simulink model "Drone_Video_Test"  (R2024a)
settings: Solver=FixedStepAuto  StartTime=0.0  StopTime=inf  RelTol=1e-3
undefined symbols (not defined in the file or in its folder): VideoDirection
settings Model: Creator=Sasha  LastModifiedBy=Sasha

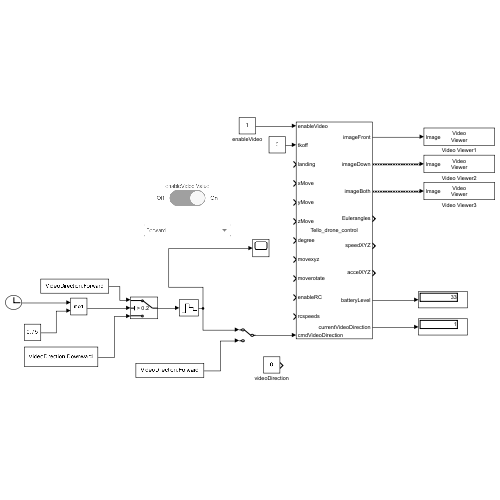
[thumbnail: Simulink's stored preview of the top-level diagram]
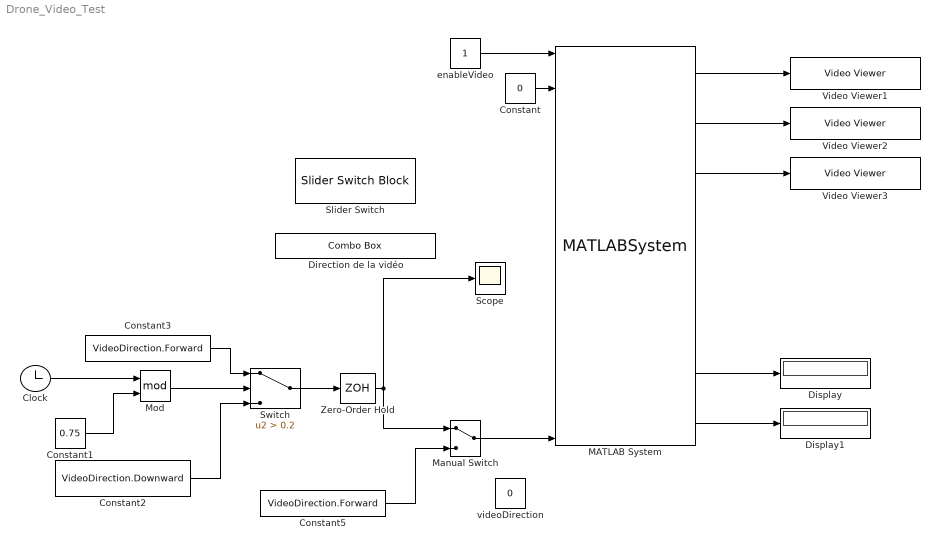
== system Drone_Video_Test ==
  Clock : Clock
  Constant : Constant  Value=0
  Constant1 : Constant  Value=0.75
  Constant2 : Constant  Value=VideoDirection.Downward
  Constant3 : Constant  Value=VideoDirection.Forward
  Constant5 : Constant  Value=VideoDirection.Forward
  Direction de la vidéo : ComboBox  LabelPosition=Hide  SelectedLabel=Forward  UseEnumeratedDataType=on  EnumeratedDataType=VideoDirection
      settings: Values={{'Forward', 'Downward', 'Both'}, [0 1 2]}
  Display : Display
  Display1 : Display
  MATLAB System : MATLABSystem  System=Tello_drone_control  droneIP=127.0.0.1  SimulateUsing=Interpreted execution
      mask Type: Tello_drone_control
      mask Display:
      | disp('Tello_drone_control');
      | port_label('input',1,'enableVideo');
      | port_label('input',2,'tkoff');
      | port_label('input',3,'landing');
      | port_label('input',4,'xMove');
      | port_label('input',5,'yMove');
      | port_label('input',6,'zMove');
      | port_label('input',7,'degree');
      | port_label('input',8,'movexyz');
      | port_label('input',9,'moverotate');
      | port_label('input',10,'enableRC');
      | port_label('input',11,'rcspeeds');
      | port_label('input',12,'cmdVideoDirection');
      | port_label('output',1,'imageFront');
      | port_label('output',2,'imageDown');
      | port_label('output',3,'imageBoth');
      | port_label('output',4,'Eulerangles');
      | port_label('output',5,'speedXYZ');
      | port_label('output',6,'accelXYZ');
      | port_label('output',7,'batteryLevel');
      | port_label('output',8,'currentVideoDirection');
  Manual Switch : ManualSwitch
  Mod : Math  Operator=mod
  Scope : Scope
  Slider Switch : SliderSwitchBlock
      settings: Values={{'Off', 'On'}, [0 1]}
  Switch : Switch  Criteria=u2 > Threshold  Threshold=0.2  SaturateOnIntegerOverflow=off  InputSameDT=off
  Video Viewer1 : VideoViewer  FigPos=[754.333333333333 474 749.333333333333 371.333333333333]
  Video Viewer2 : VideoViewer  FigPos=[754.333333333333 951.333333333333 749.333333333333 371.333333333333]
  Video Viewer3 : VideoViewer  FigPos=[128.333333333333 1165.33333333333 1080.66666666667 580]
  Zero-Order Hold : ZeroOrderHold  SampleTime=-1
  enableVideo : Constant
  videoDirection : Constant  Value=0
  wires:
  enableVideo/1 -> MATLAB System/1
  MATLAB System/1 -> Video Viewer1/1
  MATLAB System/2 -> Video Viewer2/1
  MATLAB System/3 -> Video Viewer3/1
  MATLAB System/7 -> Display/1
  Constant/1 -> MATLAB System/2
  MATLAB System/8 -> Display1/1
  Constant1/1 -> Mod/2
  Mod/1 -> Switch/2
  Constant2/1 -> Switch/3
  Constant3/1 -> Switch/1
  Switch/1 -> Zero-Order Hold/1
  Zero-Order Hold/1 -> Scope/1, Manual Switch/1
  Clock/1 -> Mod/1
  Manual Switch/1 -> MATLAB System/12
  Constant5/1 -> Manual Switch/2
